simulink model "Copy_of_EIRSAT_ADCS"  (R2014a)
settings: Solver=ode45  SolverMode=SingleTasking  StartTime=0.0  StopTime=5900*5  FixedStep=1e-9  RelTol=1e-6
values from neighbouring files (symbols this model uses):
  adr = ADRblockGen(w,m,3)    [Control_mission_def.m]    (also in CubeSimSetUp.m; Example__simulaltion.m; Example_simulaltion.m; WBC_setup.m)
  adr2 = ADRblockGen(wo2,I(2,2),3)    [CubeQuat_setup.m]    (also in WBC_setup.m = ADRblockGen(w2,m,3))
  aerodrag_A_d = 0.2*0.1*sqrt(2)    [Satellite_Setup_Sun_Pointing.m]    (also in Satellite_setup_ZenithPointing.m; WS_20_09_2017.mat = 0.0282842712475; WS_25_09_2017.mat = 0.0282842712475; WS_29_09_2017.mat = 0.0282842712475)
  aerodrag_c_p = 0.02*[1;1;1]    [Satellite_Setup_Sun_Pointing.m]    (also in Satellite_setup_ZenithPointing.m; WS_20_09_2017.mat = [0.02 0.02 0.02]; WS_25_09_2017.mat = [0.02 0.02 0.02]; WS_29_09_2017.mat = [0.02 0.02 0.02])
  distrej = 0    [Control_mission_def.m]    (also in CubeSimSetUp.m; Example__simulaltion.m; Example_simulaltion.m; WBC_setup.m = 1)
  I = diag(I_mom) + [0 I_prd(1) I_prd(2); I_prd(1) 0 I_prd(3); I_prd(2) I_prd(3) 0]    [CubeQuat_setup.m]    (also in CubeSatModel.m = reshape(I,3,3); CubeSatSfun.m = block.DialogPrm(2).Data; CubeSimSetUp.m = diag([Ixx;Iyy;Izz]); Satellite_Setup.m = diag([Ixx;Iyy;Izz]))
  igrf_G = [-29619.4 -3401.55 3349 4078.8125 -1723.05 1043.83125 2118.1875 1226.671875 474.8046875 -469.10703125 930.012890625 -1452.42753906 ... (182 elements, 13x14)]    [WS_20_09_2017.mat]    (also in WS_25_09_2017.mat; WS_29_09_2017.mat)
  igrf_H = [0 0 0 0 0 0 0 0 0 0 0 0 ... (182 elements, 13x14)]    [WS_20_09_2017.mat]    (also in WS_25_09_2017.mat; WS_29_09_2017.mat)
  igrf_L = 10    [Satellite_Setup_Sun_Pointing.m]    (also in Satellite_setup_ZenithPointing.m; WS_20_09_2017.mat; WS_25_09_2017.mat; WS_29_09_2017.mat)
  igrf_tol = 1e-9    (= 1e-09)    [Satellite_Setup_Sun_Pointing.m]    (also in Satellite_setup_ZenithPointing.m; WS_20_09_2017.mat; WS_25_09_2017.mat; WS_29_09_2017.mat)
  k = 1e-9    (= 1e-09)    [Control_mission_def.m]    (also in CubeSimSetUp.m = 1e-06; Example__simulaltion.m; Example_simulaltion.m = 5e-08; WBC_setup.m = 5e-09)
  k2 = 10    [CubeQuat_setup.m]    (also in WBC_setup.m = 5e-09; WS_20_09_2017.mat = 5e-09; WS_25_09_2017.mat = 5e-09; WS_29_09_2017.mat = 1.56433333333e-08)
  k_bd = 1e-12    [WS_20_09_2017.mat]    (also in WS_25_09_2017.mat)
  kd = 6e-4    (= 0.0006)    [Control_mission_def.m]    (also in CubeQuat_setup.m = 2*sqrt(I(1,1))*sqrt(kp); CubeSimSetUp.m; Example__simulaltion.m; Example_simulaltion.m)
  kp = 5e-9    (= 5e-09)    [Control_mission_def.m]    (also in CubeQuat_setup.m = 40; CubeSimSetUp.m; Example__simulaltion.m; Example_simulaltion.m)
  mass = 15    [CubeQuat_setup.m]    (also in CubeSimSetUp.m = 2.6; Satellite_Setup.m = 2.6; Satellite_Setup_Sun_Pointing.m = 2.6; Satellite_setup_ZenithPointing.m = 2.6)
  nA = [nAx;nAy;nAz]    [Control_mission_def.m]    (also in WS_20_09_2017.mat = [0.48 0.48 0.48]; WS_25_09_2017.mat = [0.48 0.48 0.48]; WS_29_09_2017.mat = [0.48 0.48 0.48])
  omega_orbit = [0;-7.67/(401.1+6371);0]    [CubeQuat_setup.m]    (also in CubeSatModel.m = inputs(28:30); CubeSatSfun.m = block.DialogPrm(3).Data; CubeSimSetUp.m; Satellite_Setup.m)
  q_ref = q_3_ref    [Control_mission_def.m]    (also in CubeSimSetUp.m = angle2quat(0,0,0,'XYZ'); Example__simulaltion.m; Example_simulaltion.m; WS_20_09_2017.mat = [0.707106781187 0.707106781187 0 0])
  x_0 = [0,0,0,1,0,0,0]    [CubeQuat_setup.m]    (also in CubeSimSetUp.m = [wb_bi_init;qb_o_init;qb_i_init;qo_i_init;long_init;lat_init; Example__simulaltion.m = transpose([wb_bi_init,qb_i_init]); Example_simulaltion.m = transpose([wb_bi_init,qb_i_init]); Satellite_Setup.m = transpose([wb_bi_init,qb_i_init]))
  x_orbit_init = [long_init,lat_init,altitude,qb_o_init,qo_i_init]    [Example__simulaltion.m]    (also in Example_simulaltion.m; Satellite_Setup.m; Satellite_Setup_Sun_Pointing.m; Satellite_setup_ZenithPointing.m)
undefined symbols (not defined in the file or in its folder): i_coil, m_coil, sfunxyz, SkewSym, T_act
libraries: cstblocks x24, aerolibtransform2 x7, vrlib x6
(part 1 of 2)
settings Model: Creator=JoeT  LastModifiedBy=Daire
settings OptimizationCC: BlockReduction=off  BooleanDataType=off
settings DebuggingCC: SaveWithParameterizedLinksMsg=none  UnderspecifiedInitializationDetection=Classic  SignalResolutionControl=TryResolveAllWithWarning  SolverPrmCheckMsg=none
settings HardwareCC: TargetUnknown=on

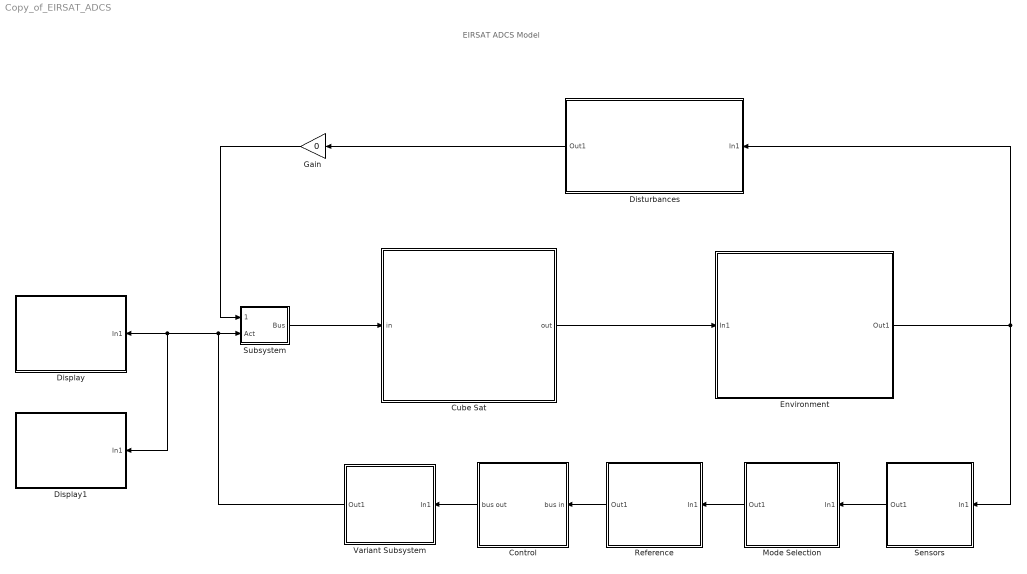
== system Copy_of_EIRSAT_ADCS ==
  note: EIRSAT ADCS Model
  Control : Subsystem  Variant=on
  Cube Sat : Subsystem
  Display : Subsystem
  Display1 : Subsystem
  Disturbances : Subsystem
  Environment : Subsystem
  Gain : Gain  Gain=0
  Mode Selection : Subsystem
  Reference : Subsystem
  Sensors : Subsystem
  Subsystem : Subsystem
  Variant Subsystem : Subsystem  Variant=on
  wires:
  Mode Selection/1(Out1) -> Reference/1(In1)
  Sensors/1(Out1) -> Mode Selection/1(In1)
  Reference/1(Out1) -> Control/1(bus in)
  Control/1(bus out) -> Variant Subsystem/1(In1)
  Disturbances/1(Out1) -> Gain/1
  Cube Sat/1(out) -> Environment/1(In1)
  Environment/1(Out1) -> Sensors/1(In1), Disturbances/1(In1)
  Variant Subsystem/1(Out1) -> Subsystem/2(Act), Display1/1(In1), Display/1(In1)
  Subsystem/1(Bus) -> Cube Sat/1(in)
  Gain/1 -> Subsystem/1(Disturb)

== system Copy_of_EIRSAT_ADCS/Control ==
  note: 1) Only subsystems can be added as variant choices at this level
      | 2) Blocks cannot be connected at this level as connectivity is
      | automatically determined at simulation, based on the active variant
  bus in : Inport
  B dot : Subsystem  VariantControl=CtrlType==4
  PD : Subsystem  VariantControl=CtrlType==2
  PD Zenith : Subsystem  VariantControl=CtrlType==3
  WBC : Subsystem  VariantControl=CtrlType==1
  WBC detumble : Subsystem  VariantControl=CtrlType==5
  no control : Subsystem  VariantControl=CtrlType==0
  bus out : Outport

== system Copy_of_EIRSAT_ADCS/Cube Sat ==
  in : Inport
  Bus Creator : BusCreator  Inputs=8
  Bus Selector1 : BusSelector  OutputSignals=T_total,T_act
  Constant : Constant  Value=omega_orbit
  Constant1 : Constant  Value=[0;0;0]
  Gain : Gain
  Gain1 : Gain
  Level-2 MATLAB S-Function : M-S-Function  FunctionName=OrbitSfun  Parameters=x_orbit_init,omega_orbit  mask{Parameter1=x_orbit_init, Parameter2=omega_orbit}
      mask prompts: Parameter1 "Initial orbit param"; Parameter2 "orbit angular velocity"
      mask DialogControl Control8 Prompt: Orbit properties
      mask Display:
      | disp('Orbital Parameters')
      | port_label('input',1,'ang vel')
      | port_label('output',1,'LLA')
      | port_label('output',2,'qb_o')
      | port_label('output',3,'qo_i')
  Satellite Dyn : M-S-Function  FunctionName=CubeSatSfun  Parameters=x_0,I  mask{Parameter2=x_0, Parameter3=I}
      mask prompts: Parameter2 "x_0"; Parameter3 "I"
      mask DialogControl DescTextVar Prompt: Model of a rigid CubeSat. Model takes Torque about each axis as an input. The first output is the angular velocity of the sat wrt an inertial frame. The second output is the quaternion which represents the rotation between inertial and body fixed frames
      mask Display:
      | disp('Cube Sat Model')
      | port_label('input',1,'Torq')
      | port_label('output',1,'Ang Vel')
      | port_label('output',2,'Quat')
  Scope : Scope
      settings: SaveName=ScopeData15
  out : Outport
  wires:
  Bus Selector1/1 -> Gain/1  "<T_total>"
  Satellite Dyn/1 -> Level-2 MATLAB S-Function/1, Bus Creator/1  "omega_b_inert"
  Gain/1 -> Satellite Dyn/1, Scope/1
  Satellite Dyn/2 -> Bus Creator/2  "qb_i"
  Level-2 MATLAB S-Function/1 -> Bus Creator/3  "LongLatAlt"
  Level-2 MATLAB S-Function/2 -> Bus Creator/4  "qb_o"
  Level-2 MATLAB S-Function/3 -> Bus Creator/5  "qo_i"
  Constant/1 -> Bus Creator/7  "omega_orbit"
  Bus Selector1/2 -> Gain1/1  "<T_act>"
  Gain1/1 -> Bus Creator/6  "T_ctrlr"
  Constant1/1 -> Bus Creator/8  "B_i"
  in/1 -> Bus Selector1/1
  Bus Creator/1 -> out/1

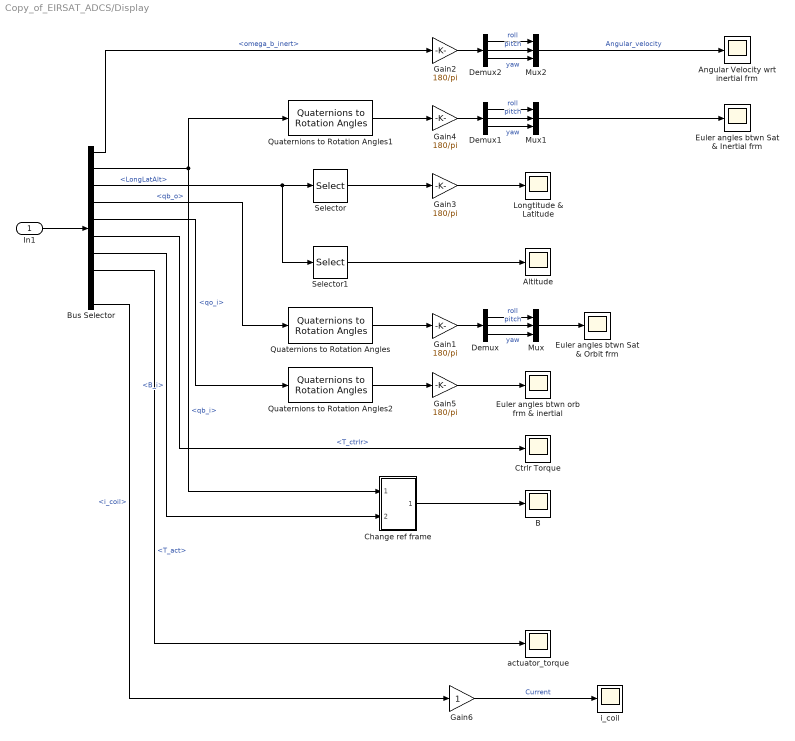
== system Copy_of_EIRSAT_ADCS/Display ==
  In1 : Inport
  Altitude : Scope
  Angular Velocity wrt inertial frm : Scope
      settings: ShowLegends=on  TimeRange=5445.680459835854  YMin=-0.3  YMax=1.1  SaveName=ScopeData5
  B : Scope
  Bus Selector : BusSelector  OutputSignals=Actual_Values.omega_b_inert,Actual_Values.qb_i,Actual_Values.LongLatAlt,Actual_Values.qb_o,Actual_Values.qo_i,Actual_Values.T_ctrlr,Actual_Values.B_i,T_act,q_ref,i_coil
  Change ref frame : Subsystem
  Ctrlr Torque : Scope
      settings: YMin=-5e-11  YMax=1.75e-10
  Demux : Demux  Outputs=3
  Demux1 : Demux  Outputs=3
  Demux2 : Demux  Outputs=3
  Euler angles btwn Sat & Inertial frm : Scope
      settings: ShowLegends=on  TimeRange=5655.978629419876  YMin=-3  YMax=4  SaveName=ScopeData8
  Euler angles btwn Sat & Orbit frm : Scope
      settings: ShowLegends=on  TimeRange=5445.680459835854  YMax=0.25
  Euler angles btwn orb frm & inertial : Scope
      settings: YMin=-200  YMax=100
  Gain{1..5} (5 alike) : Gain  Gain=180/pi
  Gain6 : Gain
  Longtitude & Latitude : Scope
  Mux : Mux  Inputs=3
  Mux1 : Mux  Inputs=3
  Mux2 : Mux  Inputs=3
  Quaternions to Rotation Angles : aerolibtransform2/Quaternions to Rotation Angles  rotationOrder=XYZ
  Quaternions to Rotation Angles1 : aerolibtransform2/Quaternions to Rotation Angles  rotationOrder=XYZ
  Quaternions to Rotation Angles2 : aerolibtransform2/Quaternions to Rotation Angles  rotationOrder=XYZ
  Selector : Selector  InputPortWidth=3  Indices=[1 2]
  Selector1 : Selector  InputPortWidth=3  Indices=[3]
  actuator_torque : Scope
      settings: YMin=-3.5e-09  YMax=2e-09
  i_coil : Scope
      settings: TimeRange=5445.680459835854  YMin=-0.001  YMax=0.0005  SaveName=ScopeData9
  wires:
  In1/1 -> Bus Selector/1
  Bus Selector/6 -> Ctrlr Torque/1  "<T_ctrlr>"
  Bus Selector/4 -> Quaternions to Rotation Angles/1  "<qb_o>"
  Bus Selector/1 -> Gain2/1  "<omega_b_inert>"
  Quaternions to Rotation Angles/1 -> Gain1/1
  Gain1/1 -> Demux/1
  Selector/1 -> Gain3/1
  Gain3/1 -> Longtitude & Latitude/1
  Bus Selector/2 -> Change ref frame/1(In1), Quaternions to Rotation Angles1/1  "<qb_i>"
  Quaternions to Rotation Angles1/1 -> Gain4/1
  Selector1/1 -> Altitude/1
  Bus Selector/5 -> Quaternions to Rotation Angles2/1  "<qo_i>"
  Quaternions to Rotation Angles2/1 -> Gain5/1
  Bus Selector/3 -> Selector1/1, Selector/1  "<LongLatAlt>"
  Bus Selector/8 -> actuator_torque/1  "<T_act>"
  Bus Selector/10 -> Gain6/1  "<i_coil>"
  Gain5/1 -> Euler angles btwn orb frm & inertial/1
  Demux/1 -> Mux/1  "roll"
  Demux/2 -> Mux/2  "pitch"
  Demux/3 -> Mux/3  "yaw"
  Mux/1 -> Euler angles btwn Sat & Orbit frm/1
  Demux1/1 -> Mux1/1  "roll"
  Demux1/2 -> Mux1/2  "pitch"
  Demux1/3 -> Mux1/3  "yaw"
  Gain4/1 -> Demux1/1
  Demux2/1 -> Mux2/1  "roll"
  Demux2/2 -> Mux2/2  "pitch"
  Demux2/3 -> Mux2/3  "yaw"
  Gain2/1 -> Demux2/1
  Mux2/1 -> Angular Velocity wrt inertial frm/1  "Angular_velocity"
  Gain6/1 -> i_coil/1  "Current"
  Mux1/1 -> Euler angles btwn Sat & Inertial frm/1
  Bus Selector/7 -> Change ref frame/2(In2)  "<B_i>"
  Change ref frame/1(Out1) -> B/1

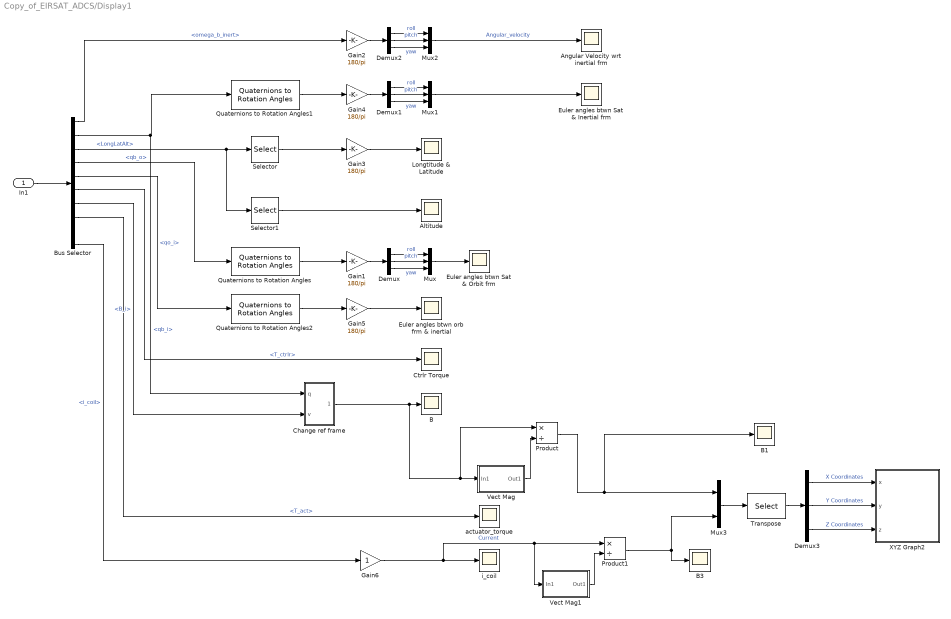
== system Copy_of_EIRSAT_ADCS/Display1 ==
  In1 : Inport
  Altitude : Scope
  Angular Velocity wrt inertial frm : Scope
      settings: ShowLegends=on  TimeRange=5445.680459835854  YMin=-0.3  YMax=1.1  SaveName=ScopeData5
  B : Scope
      settings: YMin=-2.25e-05  YMax=1.25e-05
  B1 : Scope
      settings: YMin=-0.9  YMax=0.5  SaveName=ScopeData3
  B3 : Scope
      settings: YMin=-1  YMax=0.2  SaveName=ScopeData6
  Bus Selector : BusSelector  OutputSignals=Actual_Values.omega_b_inert,Actual_Values.qb_i,Actual_Values.LongLatAlt,Actual_Values.qb_o,Actual_Values.qo_i,Actual_Values.T_ctrlr,Actual_Values.B_i,T_act,q_ref,i_coil
  Change ref frame : Subsystem
  Ctrlr Torque : Scope
      settings: YMin=-5e-11  YMax=1.75e-10
  Demux : Demux  Outputs=3
  Demux1 : Demux  Outputs=3
  Demux2 : Demux  Outputs=3
  Demux3 : Demux  Outputs=[2 2 2]
  Euler angles btwn Sat & Inertial frm : Scope
      settings: ShowLegends=on  TimeRange=5655.978629419876  YMin=-3  YMax=4  SaveName=ScopeData8
  Euler angles btwn Sat & Orbit frm : Scope
      settings: ShowLegends=on  TimeRange=5445.680459835854  YMax=0.25
  Euler angles btwn orb frm & inertial : Scope
      settings: YMin=-200  YMax=100
  Gain{1..5} (5 alike) : Gain  Gain=180/pi
  Gain6 : Gain
  Longtitude & Latitude : Scope
  Mux : Mux  Inputs=3
  Mux1 : Mux  Inputs=3
  Mux2 : Mux  Inputs=3
  Mux3 : Mux  Inputs=2
  Product : Product  Inputs=*/
  Product1 : Product  Inputs=*/
  Quaternions to Rotation Angles : aerolibtransform2/Quaternions to Rotation Angles  rotationOrder=XYZ
  Quaternions to Rotation Angles1 : aerolibtransform2/Quaternions to Rotation Angles  rotationOrder=XYZ
  Quaternions to Rotation Angles2 : aerolibtransform2/Quaternions to Rotation Angles  rotationOrder=XYZ
  Selector : Selector  InputPortWidth=3  Indices=[1 2]
  Selector1 : Selector  InputPortWidth=3  Indices=[3]
  Transpose : Selector  InputPortWidth=3*2  Indices=reshape(reshape(1:3*2,3,2)',3*2,1)
  Vect Mag : Subsystem
  Vect Mag1 : Subsystem
  XYZ Graph2 : Subsystem  LoadFcn=sfunxyz([],[],[],'LoadBlock')  StartFcn=sfunxyz([],[],[],'Start')  StopFcn=sfunxyz([],[],[],'Stop')  mask(XYZ multiscope){np=2, xlim=[-1 1], ylim=[-1 1], zlim=[-1 1], cp=[3 2 1], gd=on, st=0.1}
      mask prompts: np "Number of lines"; xlim "[xmin xmax]"; ylim "[ymin ymax]"; zlim "[zmin zmax]"; cp "Camera position (use [0 0 1] for 2D XY view)"; gd "Grid"; st "Sample time:"
      mask help:
      | Multidimensional XYZ scope using MATLAB graph window.
      |    X,Y,Z coordinates are respectively the first,second, and third input.
      |    Enter the number of lines, the XYZ ranges, the camera position,
      |    and the sampling time, as mask parameters.
      settings: CopyFcn=sfunxyz([],[],[],'CopyBlock')  DeleteFcn=sfunxyz([],[],[],'DeleteBlock')  NameChangeFcn=sfunxyz([],[],[],'NameChange')
      mask Help:
      | This block can be used to explore limit cycles.
      |    Look at the m-file sfunxyz.m to see how it works.
      mask Display: plot([.05 .95 .95 .05 .05],[.45 .45 .95 .95 .45], 0.5+cos(0:0.1:2*pi)*0.3,0.7+sin(0:0.1:2*pi)*0.2)
  actuator_torque : Scope
      settings: YMin=-3.5e-09  YMax=2e-09
  i_coil : Scope
      settings: TimeRange=5445.680459835854  YMin=-4.75e-06  YMax=7.5e-07  SaveName=ScopeData9
  wires:
  Change ref frame/1(Out1) -> Product/1, Vect Mag/1(In1), B/1
  Bus Selector/7 -> Change ref frame/2(v)  "<B_i>"
  Mux1/1 -> Euler angles btwn Sat & Inertial frm/1
  Gain6/1 -> Product1/1, Vect Mag1/1(In1), i_coil/1  "Current"
  Mux2/1 -> Angular Velocity wrt inertial frm/1  "Angular_velocity"
  Gain2/1 -> Demux2/1
  Demux2/3 -> Mux2/3  "yaw"
  Demux2/2 -> Mux2/2  "pitch"
  Demux2/1 -> Mux2/1  "roll"
  Gain4/1 -> Demux1/1
  Demux1/3 -> Mux1/3  "yaw"
  Demux1/2 -> Mux1/2  "pitch"
  Demux1/1 -> Mux1/1  "roll"
  Mux/1 -> Euler angles btwn Sat & Orbit frm/1
  Demux/3 -> Mux/3  "yaw"
  Demux/2 -> Mux/2  "pitch"
  Demux/1 -> Mux/1  "roll"
  Gain5/1 -> Euler angles btwn orb frm & inertial/1
  Bus Selector/10 -> Gain6/1  "<i_coil>"
  Bus Selector/8 -> actuator_torque/1  "<T_act>"
  Bus Selector/3 -> Selector/1, Selector1/1  "<LongLatAlt>"
  Quaternions to Rotation Angles2/1 -> Gain5/1
  Bus Selector/5 -> Quaternions to Rotation Angles2/1  "<qo_i>"
  Selector1/1 -> Altitude/1
  Quaternions to Rotation Angles1/1 -> Gain4/1
  Bus Selector/2 -> Quaternions to Rotation Angles1/1, Change ref frame/1(q)  "<qb_i>"
  Gain3/1 -> Longtitude & Latitude/1
  Selector/1 -> Gain3/1
  Gain1/1 -> Demux/1
  Quaternions to Rotation Angles/1 -> Gain1/1
  Bus Selector/1 -> Gain2/1  "<omega_b_inert>"
  Bus Selector/4 -> Quaternions to Rotation Angles/1  "<qb_o>"
  Bus Selector/6 -> Ctrlr Torque/1  "<T_ctrlr>"
  In1/1 -> Bus Selector/1
  Mux3/1 -> Transpose/1
  Transpose/1 -> Demux3/1
  Demux3/1 -> XYZ Graph2/1(x)  "X Coordinates"
  Demux3/2 -> XYZ Graph2/2(y)  "Y Coordinates"
  Demux3/3 -> XYZ Graph2/3(z)  "Z Coordinates"
  Vect Mag/1(Out1) -> Product/2
  Product/1 -> B1/1, Mux3/1
  Vect Mag1/1(Out1) -> Product1/2
  Product1/1 -> Mux3/2, B3/1

== system Copy_of_EIRSAT_ADCS/Disturbances ==
  In1 : Inport
  Bus Selector : BusSelector  OutputSignals=qb_o,omega_orbit,omega_b_inert
  Constant : Constant  Value=7.2157
  Level-2 MATLAB S-Function : M-S-Function  FunctionName=gravityGradientSfun
      mask Display:
      | disp('Gravity\n gradient')
      | port_label('input',1,'qb_o')
      | port_label('input',2,'omega orbit')
      | port_label('output',1,'T_b')
  Level-2 MATLAB S-Function1 : M-S-Function  FunctionName=aeroDragSfun  Parameters=I,mass,aerodrag_c_p,aerodrag_A_d  mask{Parameter1=I, Parameter2=mass, Parameter3=aerodrag_c_p, Parameter4=aerodrag_A_d}
      mask prompts: Parameter1 "Inertia"; Parameter2 "Mass"; Parameter3 "COP vector"; Parameter4 "Area"
      mask Display:
      | disp('Aerodynamic\n drag')
      | port_label('input',1,'qb_o')
      | port_label('input',2,'omega orbit')
      | port_label('input',3,'Local atmosph. vel')
      | port_label('output',1,'T_b')
  Sum : Sum  Inputs=|++
  Out1 : Outport
  wires:
  Level-2 MATLAB S-Function/1 -> Sum/1
  Level-2 MATLAB S-Function1/1 -> Sum/2
  In1/1 -> Bus Selector/1
  Bus Selector/1 -> Level-2 MATLAB S-Function1/1, Level-2 MATLAB S-Function/1  "<qb_o>"
  Bus Selector/2 -> Level-2 MATLAB S-Function/2, Level-2 MATLAB S-Function1/2  "<omega_orbit>"
  Constant/1 -> Level-2 MATLAB S-Function1/3
  Sum/1 -> Out1/1  "T_dst"
  Bus Selector/3 -> Level-2 MATLAB S-Function1/4  "<omega_b_inert>"

== system Copy_of_EIRSAT_ADCS/Environment ==
  In1 : Inport
  Bus Assignment : BusAssignment  AssignedSignals=B_i
  Bus Selector : BusSelector  OutputSignals=LongLatAlt
  Constant : Constant  Value=0
  Level-2 MATLAB S-Function : M-S-Function  FunctionName=IGRFSfun  Parameters=igrf_L,igrf_tol,igrf_G,igrf_H  mask{Parameter1=igrf_L, Parameter2=igrf_tol, Parameter3=igrf_G, Parameter4=igrf_H}
      mask prompts: Parameter1 "L"; Parameter2 "tolerance"; Parameter3 "G_coefs"; Parameter4 "H_coefs"
      mask Display:
      | disp('IGRF 11\n  Geomagnetic reference')
      | port_label('input',1,'LLA')
      | port_label('output',1,'real B')
  Out1 : Outport
  wires:
  In1/1 -> Bus Selector/1, Bus Assignment/1  "Dyn_out"
  Bus Selector/1 -> Level-2 MATLAB S-Function/1  "<LongLatAlt>"
  Bus Assignment/1 -> Out1/1
  Constant/1 -> Level-2 MATLAB S-Function/2  "B_real"
  Level-2 MATLAB S-Function/1 -> Bus Assignment/2  "B_real"

== system Copy_of_EIRSAT_ADCS/Mode Selection ==
  In1 : Inport
  Bus Assignment : BusAssignment  AssignedSignals=Mode
  Constant : Constant
  Out1 : Outport
  wires:
  In1/1 -> Bus Assignment/1  "Sensor_out"
  Bus Assignment/1 -> Out1/1
  Constant/1 -> Bus Assignment/2  "mode"

== system Copy_of_EIRSAT_ADCS/Reference ==
  In1 : Inport
  Bus Assignment : BusAssignment  AssignedSignals=q_ref
  Constant : Constant  Value=q_ref
  Out1 : Outport
  wires:
  In1/1 -> Bus Assignment/1
  Bus Assignment/1 -> Out1/1
  Constant/1 -> Bus Assignment/2  "q_ref"

== system Copy_of_EIRSAT_ADCS/Sensors ==
  In1 : Inport
  Bus Creator1 : BusCreator  Inputs=10
  Bus Selector : BusSelector  OutputSignals=B_i,LongLatAlt,qb_i,omega_b_inert  OutputAsBus=on
  Constant : Constant
  Constant1 : Constant  Value=[1,0,0,0]
  Constant{2..7} (6 alike) : Constant  Value=[0;0;0]
  Out1 : Outport
  wires:
  In1/1 -> Bus Creator1/1, Bus Selector/1  "Actual_Values"
  Bus Creator1/1 -> Out1/1
  Bus Selector/1 -> Bus Creator1/2  "Sensor_Values"
  Constant/1 -> Bus Creator1/3  "Mode"
  Constant1/1 -> Bus Creator1/4  "q_ref"
  Constant2/1 -> Bus Creator1/5  "m_b"
  Constant3/1 -> Bus Creator1/6  "m_coil"
  Constant4/1 -> Bus Creator1/7  "T_act"
  Constant5/1 -> Bus Creator1/8  "i_coil"
  Constant6/1 -> Bus Creator1/9  "T_total"
  Constant7/1 -> Bus Creator1/10  "T_ctrlr"

== system Copy_of_EIRSAT_ADCS/Subsystem ==
  Disturb : Inport
  Act : Inport  Port=2
  Bus Assignment : BusAssignment  AssignedSignals=T_total
  Bus Selector1 : BusSelector  OutputSignals=T_act
  Sum : Sum  Inputs=++|
  Bus : Outport
  wires:
  Disturb/1 -> Sum/2
  Act/1 -> Bus Assignment/1, Bus Selector1/1
  Sum/1 -> Bus Assignment/2  "T_total"
  Bus Selector1/1 -> Sum/1  "<T_act>"
  Bus Assignment/1 -> Bus/1

== system Copy_of_EIRSAT_ADCS/Variant Subsystem ==
  note: 1) Only subsystems can be added as variant choices at this level
      | 2) Blocks cannot be connected at this level as connectivity is
      | automatically determined at simulation, based on the active variant
  In1 : Inport
  2 coil dipole : Subsystem  VariantControl=ActType==5
  3 coil dipole : Subsystem  VariantControl=ActType==4
  Ideal Torque : Subsystem  VariantControl=ActType==1
  No Torque : Subsystem  VariantControl=ActType==0
  Three Axis MagTorq : Subsystem  VariantControl=ActType==2
  Two Axis MagTorq : Subsystem  VariantControl=ActType==3
  Out1 : Outport

== system Copy_of_EIRSAT_ADCS/Control/B dot ==
  bus in : Inport
  Bus Creator : BusCreator  Inputs=2
  Bus Selector : BusSelector  OutputSignals=signal1.Sensor_out.Sensor_Values.qb_i,q_ref,signal1.Sensor_out.Sensor_Values.omega_b_inert,signal1.Sensor_out.Sensor_Values.B_real,signal1.Sensor_out.Actual_Values.Dyn_out.qb_o
  Derivative : Derivative
  Gain : Gain  Gain=-k_bd
  bus out : Outport
  wires:
  Bus Creator/1 -> bus out/1
  bus in/1 -> Bus Creator/1, Bus Selector/1  "ref_out"
  Bus Selector/4 -> Derivative/1  "<B_real>"
  Derivative/1 -> Gain/1
  Gain/1 -> Bus Creator/2  "T_ctrlr"

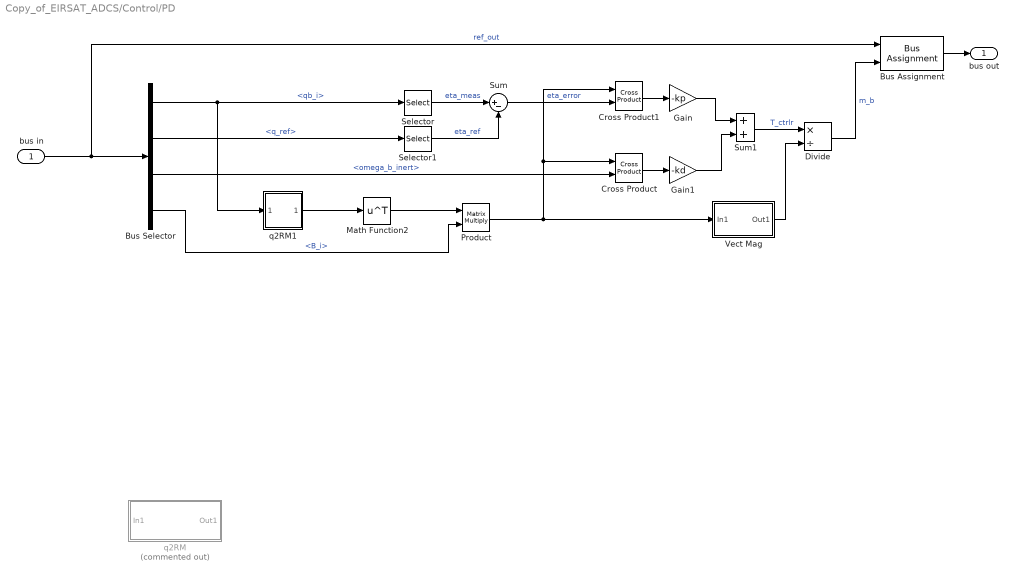
== system Copy_of_EIRSAT_ADCS/Control/PD ==
  bus in : Inport
  Bus Assignment : BusAssignment  AssignedSignals=m_b
  Bus Selector : BusSelector  OutputSignals=Sensor_Values.qb_i,q_ref,Sensor_Values.omega_b_inert,Sensor_Values.B_i
  Cross Product : vrlib/Utilities/Cross Product
  Cross Product1 : vrlib/Utilities/Cross Product
  Divide : Product  Inputs=*/
  Gain : Gain  Gain=-kp
  Gain1 : Gain  Gain=-kd
  Math Function2 : Math  Operator=transpose  SaturateOnIntegerOverflow=on
  Product : Product  Multiplication=Matrix(*)
  Selector : Selector  InputPortWidth=4  Indices=[2 3 4]
  Selector1 : Selector  InputPortWidth=4  Indices=[2 3 4]
  Sum : Sum  Inputs=|+-
  Sum1 : Sum
  Vect Mag : Subsystem
  q2RM : Subsystem  Commented=on
  q2RM1 : Subsystem
  bus out : Outport
  wires:
  bus in/1 -> Bus Assignment/1, Bus Selector/1  "ref_out"
  Bus Selector/2 -> Selector1/1  "<q_ref>"
  Selector/1 -> Sum/1  "eta_meas"
  Selector1/1 -> Sum/2  "eta_ref"
  Gain/1 -> Sum1/1
  Gain1/1 -> Sum1/2
  Bus Assignment/1 -> bus out/1
  Product/1 -> Cross Product1/1, Cross Product/1, Vect Mag/1(In1)
  Vect Mag/1(Out1) -> Divide/2
  Sum/1 -> Cross Product1/2  "eta_error"
  Bus Selector/1 -> q2RM1/1(In1), Selector/1  "<qb_i>"
  Cross Product1/1 -> Gain/1
  Cross Product/1 -> Gain1/1
  Divide/1 -> Bus Assignment/2  "m_b"
  Bus Selector/4 -> Product/2  "<B_i>"
  Math Function2/1 -> Product/1
  q2RM1/1(Out1) -> Math Function2/1
  Sum1/1 -> Divide/1  "T_ctrlr"
  Bus Selector/3 -> Cross Product/2  "<omega_b_inert>"

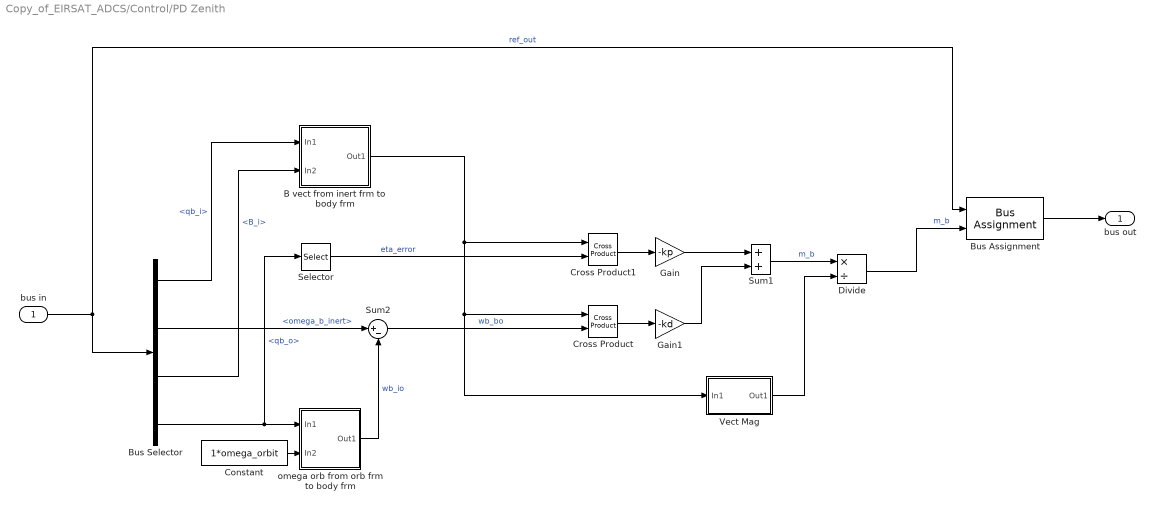
== system Copy_of_EIRSAT_ADCS/Control/PD Zenith ==
  bus in : Inport
  B vect from inert frm to body frm : Subsystem
  Bus Assignment : BusAssignment  AssignedSignals=m_b
  Bus Selector : BusSelector  OutputSignals=Sensor_Values.qb_i,Sensor_Values.omega_b_inert,Sensor_Values.B_i,Actual_Values.qb_o
  Constant : Constant  Value=1*omega_orbit
  Cross Product : vrlib/Utilities/Cross Product
  Cross Product1 : vrlib/Utilities/Cross Product
  Divide : Product  Inputs=*/
  Gain : Gain  Gain=-kp
  Gain1 : Gain  Gain=-kd
  Selector : Selector  InputPortWidth=4  Indices=[2 3 4]
  Sum1 : Sum
  Sum2 : Sum  Inputs=|+-
  Vect Mag : Subsystem
  omega orb from orb frm to body frm : Subsystem
  bus out : Outport
  wires:
  Divide/1 -> Bus Assignment/2  "m_b"
  Cross Product1/1 -> Gain/1
  Cross Product/1 -> Gain1/1
  Selector/1 -> Cross Product1/2  "eta_error"
  Sum1/1 -> Divide/1  "m_b"
  Sum2/1 -> Cross Product/2  "wb_bo"
  Vect Mag/1(Out1) -> Divide/2
  Bus Assignment/1 -> bus out/1
  Gain1/1 -> Sum1/2
  Gain/1 -> Sum1/1
  bus in/1 -> Bus Assignment/1, Bus Selector/1  "ref_out"
  Bus Selector/2 -> Sum2/1  "<omega_b_inert>"
  Bus Selector/4 -> Selector/1, omega orb from orb frm to body frm/1(In1)  "<qb_o>"
  Constant/1 -> omega orb from orb frm to body frm/2(In2)
  omega orb from orb frm to body frm/1(Out1) -> Sum2/2  "wb_io"
  B vect from inert frm to body frm/1(Out1) -> Vect Mag/1(In1), Cross Product/1, Cross Product1/1
  Bus Selector/1 -> B vect from inert frm to body frm/1(In1)  "<qb_i>"
  Bus Selector/3 -> B vect from inert frm to body frm/2(In2)  "<B_i>"

== system Copy_of_EIRSAT_ADCS/Control/WBC ==
  bus in : Inport
  Bus Assignment : BusAssignment  AssignedSignals=T_ctrlr
  Bus Selector : BusSelector  OutputSignals=q_ref,Sensor_Values.qb_i,Actual_Values.T_ctrlr,Sensor_Values.B_i
  Demux1 : Demux  Outputs=3
  Demux3 : Demux  Outputs=3
  Demux4 : Demux  Outputs=3
  Mux4 : Mux  Inputs=3
  Selector : Selector  InputPortWidth=4  Indices=[2 3 4]
  Selector1 : Selector  InputPortWidth=4  Indices=[2 3 4]
  WBC_x : Subsystem
  WBC_y : Subsystem
  WBC_z : Subsystem
  bus out : Outport
  wires:
  Demux3/3 -> WBC_z/2(x_1)
  WBC_y/1(T) -> Mux4/2
  Mux4/1 -> Bus Assignment/2  "T_ctrlr"
  WBC_z/1(T) -> Mux4/3
  WBC_x/1(T) -> Mux4/1
  Demux3/2 -> WBC_y/2(x_1)
  Demux3/1 -> WBC_x/2(x_1)
  Bus Selector/3 -> Demux1/1  "<T_ctrlr>"
  Demux1/1 -> WBC_x/3(T_meas)
  Demux1/2 -> WBC_y/3(T_meas)
  Demux1/3 -> WBC_z/3(T_meas)
  Demux4/1 -> WBC_x/1(x_0_ref)
  Demux4/3 -> WBC_z/1(x_0_ref)
  Demux4/2 -> WBC_y/1(x_0_ref)
  Selector1/1 -> Demux3/1
  bus in/1 -> Bus Assignment/1, Bus Selector/1  "ref_out"
  Bus Selector/1 -> Selector/1  "<q_ref>"
  Bus Selector/2 -> Selector1/1  "<qb_i>"
  Bus Assignment/1 -> bus out/1
  Selector/1 -> Demux4/1

== system Copy_of_EIRSAT_ADCS/Control/WBC detumble ==
  bus in : Inport
  Bus Creator : BusCreator  Inputs=2
  Bus Selector : BusSelector  OutputSignals=q_ref,signal1.Sensor_out.Sensor_values.omega_b_inert,signal1.Sensor_out.Enviro_out.Dyn_out.T_ctrlr
  Demux1 : Demux  Outputs=3
  Demux3 : Demux  Outputs=3
  Demux4 : Demux  Outputs=3
  Mux4 : Mux  Inputs=3
  Quaternions to Rotation Angles : aerolibtransform2/Quaternions to Rotation Angles  Commented=on  rotationOrder=ZYX
  Vector Mag1 : Subsystem  Commented=on
  WBC_x : Subsystem
  WBC_y : Subsystem
  WBC_z : Subsystem
  bus out : Outport
  wires:
  ? -> Demux4/1
  Bus Creator/1 -> bus out/1
  Bus Selector/2 -> Demux3/1  "<omega_b_inert>"
  Bus Selector/1 -> ?  "<q_ref>"
  bus in/1 -> Bus Selector/1, Bus Creator/1  "ref_out"
  Demux4/2 -> WBC_y/1(x_0_ref)
  Demux4/3 -> WBC_z/1(x_0_ref)
  Demux4/1 -> WBC_x/1(x_0_ref)
  Demux1/3 -> WBC_z/3(T_meas)
  Demux1/2 -> WBC_y/3(T_meas)
  Demux1/1 -> WBC_x/3(T_meas)
  Bus Selector/3 -> Demux1/1  "<T_ctrlr>"
  Demux3/1 -> WBC_x/2(x_1)
  Demux3/2 -> WBC_y/2(x_1)
  WBC_x/1(T) -> Mux4/1
  WBC_z/1(T) -> Mux4/3
  Mux4/1 -> Bus Creator/2  "T_ctrlr"
  WBC_y/1(T) -> Mux4/2
  Demux3/3 -> WBC_z/2(x_1)

== system Copy_of_EIRSAT_ADCS/Control/no control ==
  bus in : Inport
  Bus : Subsystem  Commented=on
  Bus Creator : BusCreator  Inputs=2
  Constant : Constant  Value=[0;0;0]
  bus out : Outport
  wires:
  bus in/1 -> Bus Creator/1  "ref_out"
  Constant/1 -> Bus Creator/2  "T_ctrlr"
  Bus Creator/1 -> bus out/1

== system Copy_of_EIRSAT_ADCS/Display/Change ref frame ==
  In1 : Inport
  In2 : Inport  Port=2
  Math Function2 : Math  Operator=transpose  SaturateOnIntegerOverflow=on
  Product : Product  Multiplication=Matrix(*)
  q2RM1 : Subsystem
  Out1 : Outport
  wires:
  Product/1 -> Out1/1
  Math Function2/1 -> Product/1
  In2/1 -> Product/2
  q2RM1/1(Out1) -> Math Function2/1
  In1/1 -> q2RM1/1(In1)

== system Copy_of_EIRSAT_ADCS/Display1/Change ref frame ==
  q : Inport
  v : Inport  Port=2
  Math Function2 : Math  Operator=transpose  SaturateOnIntegerOverflow=on
  Product : Product  Multiplication=Matrix(*)
  q2RM1 : Subsystem
  Out1 : Outport
  wires:
  q/1 -> q2RM1/1(In1)
  q2RM1/1(Out1) -> Math Function2/1
  v/1 -> Product/2
  Math Function2/1 -> Product/1
  Product/1 -> Out1/1

== system Copy_of_EIRSAT_ADCS/Display1/Vect Mag ==
  In1 : Inport
  Math Function : Math  Operator=square  SaturateOnIntegerOverflow=on
  Sqrt : Sqrt  SaturateOnIntegerOverflow=on
  Sum2 : Sum  Inputs=+
  Out1 : Outport
  wires:
  Sqrt/1 -> Out1/1
  In1/1 -> Math Function/1
  Math Function/1 -> Sum2/1
  Sum2/1 -> Sqrt/1

== system Copy_of_EIRSAT_ADCS/Display1/Vect Mag1 ==
  In1 : Inport
  Math Function : Math  Operator=square  SaturateOnIntegerOverflow=on
  Sqrt : Sqrt  SaturateOnIntegerOverflow=on
  Sum2 : Sum  Inputs=+
  Out1 : Outport
  wires:
  Sum2/1 -> Sqrt/1
  Math Function/1 -> Sum2/1
  In1/1 -> Math Function/1
  Sqrt/1 -> Out1/1

== system Copy_of_EIRSAT_ADCS/Display1/XYZ Graph2 ==
  x : Inport
  y : Inport  Port=2
  z : Inport  Port=3
  Mux : Mux  Inputs=[np np np]
  sfunxy : S-Function  FunctionName=sfunxyz  Parameters=[xlim ylim zlim],st,np,cp,gd  EnableBusSupport=off
  wires:
  z/1 -> Mux/3
  y/1 -> Mux/2
  x/1 -> Mux/1
  Mux/1 -> sfunxy/1

== system Copy_of_EIRSAT_ADCS/Variant Subsystem/2 coil dipole ==
  In1 : Inport
  B vect from inert frm to body frm : Subsystem
  Bus Assignment : BusAssignment  AssignedSignals=m_coil,T_act,i_coil
  Bus Selector : BusSelector  OutputSignals=m_b,Sensor_Values.B_i,Sensor_Values.qb_i
  Constant : Constant  Value=nA
  Constant3 : Constant  Value=0
  Cross Product : vrlib/Utilities/Cross Product
  Divide : Product  Inputs=*/
  Mux1 : Mux  Inputs=2
  Saturation : Saturate  UpperLimit=0.24  LowerLimit=-0.24
  Selector : Selector  InputPortWidth=3  Indices=[1 2]
  Out1 : Outport
  wires:
  Saturation/1 -> Bus Assignment/2, Divide/1, Cross Product/1
  Constant/1 -> Divide/2
  Divide/1 -> Bus Assignment/4  "i_coil"
  Bus Selector/1 -> Selector/1  "<m_b>"
  Cross Product/1 -> Bus Assignment/3  "T_act"
  Bus Assignment/1 -> Out1/1
  In1/1 -> Bus Selector/1, Bus Assignment/1  "Ctrlr_out"
  Mux1/1 -> Saturation/1
  Selector/1 -> Mux1/1
  Constant3/1 -> Mux1/2
  Bus Selector/2 -> B vect from inert frm to body frm/1(B_i)  "<B_i>"
  Bus Selector/3 -> B vect from inert frm to body frm/2(q)  "<qb_i>"
  B vect from inert frm to body frm/1(B_b) -> Cross Product/2

== system Copy_of_EIRSAT_ADCS/Variant Subsystem/3 coil dipole ==
  In1 : Inport
  B vect from inert frm to body frm : Subsystem
  Bus Assignment : BusAssignment  AssignedSignals=m_coil,T_act,i_coil
  Bus Selector : BusSelector  OutputSignals=m_b,Sensor_Values.B_i,Sensor_Values.qb_i
  Constant : Constant  Value=nA
  Cross Product : vrlib/Utilities/Cross Product
  Divide : Product  Inputs=*/
  Saturation : Saturate  UpperLimit=0.24  LowerLimit=-0.24
  Out1 : Outport
  wires:
  Saturation/1 -> Bus Assignment/2, Divide/1, Cross Product/1
  Constant/1 -> Divide/2
  Divide/1 -> Bus Assignment/4  "i_coil"
  Bus Selector/1 -> Saturation/1  "<m_b>"
  Cross Product/1 -> Bus Assignment/3  "T_act"
  In1/1 -> Bus Selector/1, Bus Assignment/1  "Ctrlr_out"
  Bus Selector/2 -> B vect from inert frm to body frm/1(B_i)  "<B_i>"
  Bus Selector/3 -> B vect from inert frm to body frm/2(q)  "<qb_i>"
  B vect from inert frm to body frm/1(B_b) -> Cross Product/2
  Bus Assignment/1 -> Out1/1

== system Copy_of_EIRSAT_ADCS/Variant Subsystem/Ideal Torque ==
  In1 : Inport
  Bus Creator : BusCreator  Inputs=3
  Bus Selector : BusSelector  OutputSignals=Actual_Values.T_ctrlr
  Constant : Constant  Value=[0,0,0]
  Gain : Gain
  Out1 : Outport
  wires:
  In1/1 -> Bus Selector/1, Bus Creator/1  "Ctrlr_out"
  Bus Creator/1 -> Out1/1
  Bus Selector/1 -> Gain/1  "<T_ctrlr>"
  Gain/1 -> Bus Creator/2  "T_act"
  Constant/1 -> Bus Creator/3  "i_coil"

== system Copy_of_EIRSAT_ADCS/Variant Subsystem/No Torque ==
  In1 : Inport
  Bus Assignment : BusAssignment  AssignedSignals=T_act,m_coil,i_coil
  Constant : Constant  Value=[0;0;0]
  Out1 : Outport
  wires:
  In1/1 -> Bus Assignment/1
  Bus Assignment/1 -> Out1/1
  Constant/1 -> Bus Assignment/4, Bus Assignment/3, Bus Assignment/2

== system Copy_of_EIRSAT_ADCS/Variant Subsystem/Three Axis MagTorq ==
  In1 : Inport
  B vect from inert frm to body frm : Subsystem
  B vect from inert frm to body frm1 : Subsystem
  Bus Assignment : BusAssignment  AssignedSignals=T_act,m_coil,i_coil
  Bus Selector : BusSelector  OutputSignals=T_ctrlr,Actual_Values.B_i,Sensor_Values.B_i,Sensor_Values.qb_i
  Level-2 MATLAB S-Function : M-S-Function  FunctionName=Magtorq2Sfun  Parameters=nAx, nAy, nAz
  Out1 : Outport
  wires:
  In1/1 -> Bus Assignment/1, Bus Selector/1
  Bus Assignment/1 -> Out1/1
  Bus Selector/3 -> Level-2 MATLAB S-Function/3, B vect from inert frm to body frm1/2(B_i)  "<B_i>"
  Level-2 MATLAB S-Function/1 -> Bus Assignment/2  "T_act"
  Bus Selector/1 -> Level-2 MATLAB S-Function/1  "<T_ctrlr>"
  Bus Selector/2 -> Level-2 MATLAB S-Function/2, B vect from inert frm to body frm/2(B_i)  "<B_i>"
  Level-2 MATLAB S-Function/2 -> Bus Assignment/3  "m_coil"
  Level-2 MATLAB S-Function/3 -> Bus Assignment/4  "i_coil"
  Bus Selector/4 -> B vect from inert frm to body frm1/1(q), B vect from inert frm to body frm/1(q)  "<qb_i>"
  B vect from inert frm to body frm/1(B_b) -> ?
  B vect from inert frm to body frm1/1(B_b) -> ?

== system Copy_of_EIRSAT_ADCS/Variant Subsystem/Two Axis MagTorq ==
  In1 : Inport
  Bus Creator : BusCreator
  Bus Selector : BusSelector  OutputSignals=T_ctrlr,ref_out.Mode_select_out.Sensor_out.Enviro_out.B_real,ref_out.Mode_select_out.Sensor_out.Sensor_values.B_real
  Level-2 MATLAB S-Function : M-S-Function  FunctionName=MagtorqSfun
  Selector : Selector  InputPortWidth=3  Indices=[1 2]
  Out1 : Outport
  wires:
  In1/1 -> Bus Selector/1, Bus Creator/1
  Bus Creator/1 -> Out1/1
  Bus Selector/3 -> Level-2 MATLAB S-Function/3  "<B_real>"
  Bus Selector/1 -> Level-2 MATLAB S-Function/1  "<T_ctrlr>"
  Bus Selector/2 -> Level-2 MATLAB S-Function/2  "<B_real>"
  Level-2 MATLAB S-Function/1 -> Selector/1
  Selector/1 -> Bus Creator/2  "m_coils"
  Level-2 MATLAB S-Function/2 -> Bus Creator/3
  ? -> Bus Creator/4  "i_coil"

== system Copy_of_EIRSAT_ADCS/Control/PD/Vect Mag ==
  In1 : Inport
  Math Function : Math  Operator=square  SaturateOnIntegerOverflow=on
  Sqrt : Sqrt  SaturateOnIntegerOverflow=on
  Sum2 : Sum  Inputs=+
  Out1 : Outport
  wires:
  Sqrt/1 -> Out1/1
  In1/1 -> Math Function/1
  Math Function/1 -> Sum2/1
  Sum2/1 -> Sqrt/1

== system Copy_of_EIRSAT_ADCS/Control/PD/q2RM ==
  In1 : Inport
  Add : Sum
  Constant : Constant  Value=eye(3)
  Fcn1 : Fcn  Expr=SkewSym([u(1),u(2),u(3)])
  Gain : Gain
  Math Function : Math  Operator=square  SaturateOnIntegerOverflow=on
  Product : Product
  Selector : Selector  InputPortWidth=4  Indices=[1]
  Selector1 : Selector  InputPortWidth=4  Indices=[2 3 4]
  Sum : Sum
  Out1 : Outport
  wires:
  In1/1 -> Selector/1, Selector1/1
  Fcn1/1 -> Math Function/1, Product/2
  Selector/1 -> Product/1
  Selector1/1 -> Fcn1/1
  Product/1 -> Sum/1
  Math Function/1 -> Sum/2
  Sum/1 -> Gain/1
  Gain/1 -> Add/2
  Constant/1 -> Add/1
  Add/1 -> Out1/1

== system Copy_of_EIRSAT_ADCS/Control/PD/q2RM1 ==
  In1 : Inport
  Add : Sum
  Constant : Constant  Value=eye(3)
  Fcn : Fcn  Commented=on  Expr=SkewSym([u(1),u(2),u(3)])
  Gain : Gain  Gain=2
  Interpreted MATLAB Function : MATLABFcn  MATLABFcn=SkewSym([u(1),u(2),u(3)],1)  OutputDimensions=9
  Math Function : Math  Operator=square  SaturateOnIntegerOverflow=on
  Product : Product
  Reshape : Reshape  OutputDimensionality=Customize  OutputDimensions=[3,3]
  Selector : Selector  InputPortWidth=4  Indices=[1]
  Selector1 : Selector  InputPortWidth=4  Indices=[2 3 4]
  Sum : Sum
  Out1 : Outport
  wires:
  In1/1 -> Selector/1, Selector1/1
  Reshape/1 -> Math Function/1, Product/2
  Selector/1 -> Product/1
  Selector1/1 -> Interpreted MATLAB Function/1
  Product/1 -> Sum/1
  Math Function/1 -> Sum/2
  Sum/1 -> Gain/1
  Gain/1 -> Add/2
  Constant/1 -> Add/1
  Add/1 -> Out1/1
  Interpreted MATLAB Function/1 -> Reshape/1

== system Copy_of_EIRSAT_ADCS/Control/PD Zenith/B vect from inert frm to body frm ==
  In1 : Inport
  In2 : Inport  Port=2
  Math Function1 : Math  Operator=transpose  SaturateOnIntegerOverflow=on
  Product1 : Product  Multiplication=Matrix(*)
  q2RM2 : Subsystem
  Out1 : Outport
  wires:
  Product1/1 -> Out1/1
  q2RM2/1(Out1) -> Math Function1/1
  In1/1 -> q2RM2/1(In1)
  Math Function1/1 -> Product1/1
  In2/1 -> Product1/2

== system Copy_of_EIRSAT_ADCS/Control/PD Zenith/Vect Mag ==
  In1 : Inport
  Math Function : Math  Operator=square  SaturateOnIntegerOverflow=on
  Sqrt : Sqrt  SaturateOnIntegerOverflow=on
  Sum2 : Sum  Inputs=+
  Out1 : Outport
  wires:
  Sum2/1 -> Sqrt/1
  Math Function/1 -> Sum2/1
  In1/1 -> Math Function/1
  Sqrt/1 -> Out1/1

== system Copy_of_EIRSAT_ADCS/Control/PD Zenith/omega orb from orb frm to body frm ==
  In1 : Inport
  In2 : Inport  Port=2
  Math Function2 : Math  Operator=transpose  SaturateOnIntegerOverflow=on
  Product : Product  Multiplication=Matrix(*)
  q2RM1 : Subsystem
  Out1 : Outport
  wires:
  Product/1 -> Out1/1
  In2/1 -> Product/2
  q2RM1/1(Out1) -> Math Function2/1
  Math Function2/1 -> Product/1
  In1/1 -> q2RM1/1(In1)

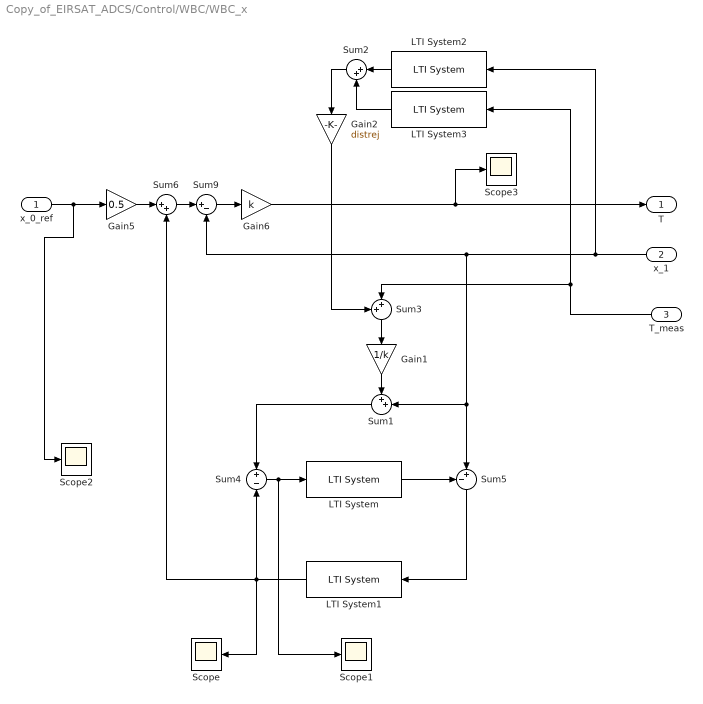
== system Copy_of_EIRSAT_ADCS/Control/WBC/WBC_x ==
  x_0_ref : Inport
  x_1 : Inport  Port=2
  T_meas : Inport  Port=3
  Gain1 : Gain  Gain=1/k
  Gain2 : Gain  Gain=distrej
  Gain5 : Gain  Gain=0.5
  Gain6 : Gain  Gain=k
  LTI System : cstblocks/LTI System  sys=G  IC=[]
  LTI System1 : cstblocks/LTI System  sys=G  IC=[]
  LTI System2 : cstblocks/LTI System  sys=adr(1)  IC=[]
  LTI System3 : cstblocks/LTI System  sys=adr(2)  IC=[]
  Scope{,1..3} (4 alike) : Scope
  Sum1 : Sum  Inputs=++|
  Sum2 : Sum  Inputs=|++
  Sum3 : Sum  Inputs=++|
  Sum4 : Sum  Inputs=+|-
  Sum5 : Sum  Inputs=-+|
  Sum6 : Sum  Inputs=|++
  Sum9 : Sum  Inputs=|+-
  T : Outport
  wires:
  Sum1/1 -> Sum4/1
  Gain1/1 -> Sum1/1
  x_1/1 -> Sum1/2, Sum5/2, Sum9/2, LTI System2/1
  Sum5/1 -> LTI System1/1
  LTI System/1 -> Sum5/1
  Sum4/1 -> Scope1/1, LTI System/1
  LTI System1/1 -> Sum4/2, Scope/1, Sum6/2
  Gain5/1 -> Sum6/1
  Gain6/1 -> Scope3/1, T/1
  Sum9/1 -> Gain6/1
  Sum6/1 -> Sum9/1
  LTI System2/1 -> Sum2/1
  LTI System3/1 -> Sum2/2
  Sum2/1 -> Gain2/1
  Sum3/1 -> Gain1/1
  Gain2/1 -> Sum3/1
  T_meas/1 -> Sum3/2, LTI System3/1
  x_0_ref/1 -> Scope2/1, Gain5/1

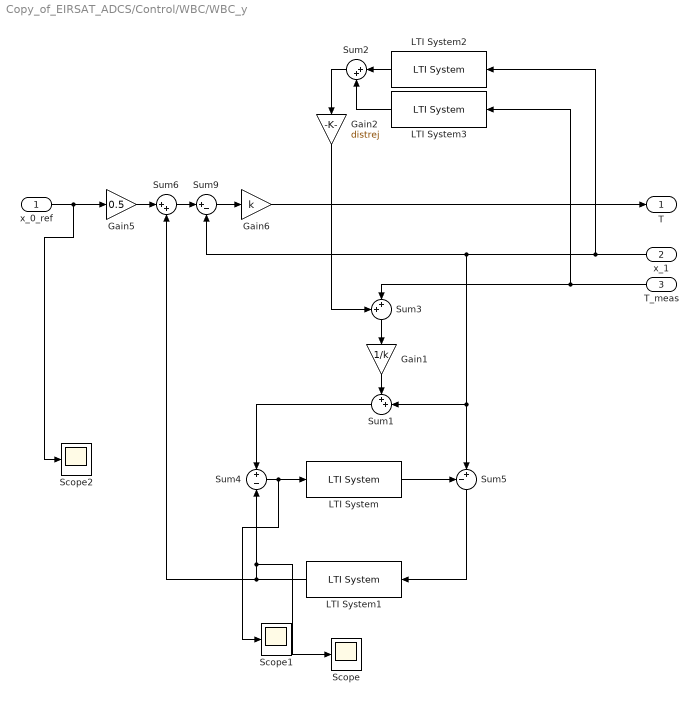
== system Copy_of_EIRSAT_ADCS/Control/WBC/WBC_y ==
  x_0_ref : Inport
  x_1 : Inport  Port=2
  T_meas : Inport  Port=3
  Gain1 : Gain  Gain=1/k
  Gain2 : Gain  Gain=distrej
  Gain5 : Gain  Gain=0.5
  Gain6 : Gain  Gain=k
  LTI System : cstblocks/LTI System  sys=G  IC=[]
  LTI System1 : cstblocks/LTI System  sys=G  IC=[]
  LTI System2 : cstblocks/LTI System  sys=adr(1)  IC=[]
  LTI System3 : cstblocks/LTI System  sys=adr(2)  IC=[]
  Scope : Scope
  Scope1 : Scope
  Scope2 : Scope
  Sum1 : Sum  Inputs=++|
  Sum2 : Sum  Inputs=|++
  Sum3 : Sum  Inputs=++|
  Sum4 : Sum  Inputs=+|-
  Sum5 : Sum  Inputs=-+|
  Sum6 : Sum  Inputs=|++
  Sum9 : Sum  Inputs=|+-
  T : Outport
  wires:
  x_0_ref/1 -> Gain5/1, Scope2/1
  T_meas/1 -> LTI System3/1, Sum3/2
  Gain2/1 -> Sum3/1
  Sum3/1 -> Gain1/1
  Sum2/1 -> Gain2/1
  LTI System3/1 -> Sum2/2
  LTI System2/1 -> Sum2/1
  Sum6/1 -> Sum9/1
  Sum9/1 -> Gain6/1
  Gain6/1 -> T/1
  Gain5/1 -> Sum6/1
  LTI System1/1 -> Sum6/2, Sum4/2, Scope/1
  Sum4/1 -> LTI System/1, Scope1/1
  LTI System/1 -> Sum5/1
  Sum5/1 -> LTI System1/1
  x_1/1 -> LTI System2/1, Sum9/2, Sum5/2, Sum1/2
  Gain1/1 -> Sum1/1
  Sum1/1 -> Sum4/1

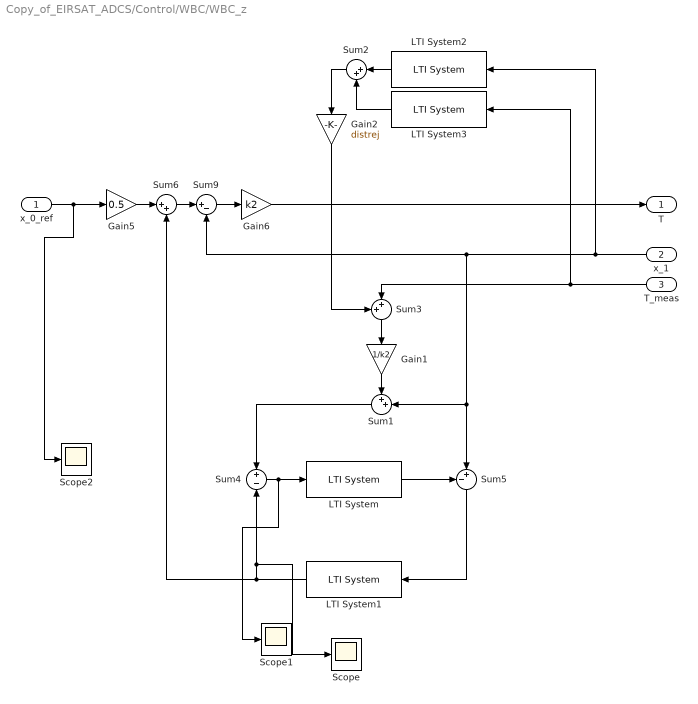
== system Copy_of_EIRSAT_ADCS/Control/WBC/WBC_z ==
  x_0_ref : Inport
  x_1 : Inport  Port=2
  T_meas : Inport  Port=3
  Gain1 : Gain  Gain=1/k2
  Gain2 : Gain  Gain=distrej
  Gain5 : Gain  Gain=0.5
  Gain6 : Gain  Gain=k2
  LTI System : cstblocks/LTI System  sys=G2  IC=[]
  LTI System1 : cstblocks/LTI System  sys=G2  IC=[]
  LTI System2 : cstblocks/LTI System  sys=adr2(1)  IC=[]
  LTI System3 : cstblocks/LTI System  sys=adr2(2)  IC=[]
  Scope : Scope
  Scope1 : Scope
  Scope2 : Scope
  Sum1 : Sum  Inputs=++|
  Sum2 : Sum  Inputs=|++
  Sum3 : Sum  Inputs=++|
  Sum4 : Sum  Inputs=+|-
  Sum5 : Sum  Inputs=-+|
  Sum6 : Sum  Inputs=|++
  Sum9 : Sum  Inputs=|+-
  T : Outport
  wires:
  Sum1/1 -> Sum4/1
  Gain1/1 -> Sum1/1
  x_1/1 -> Sum1/2, Sum5/2, Sum9/2, LTI System2/1
  Sum5/1 -> LTI System1/1
  LTI System/1 -> Sum5/1
  Sum4/1 -> Scope1/1, LTI System/1
  LTI System1/1 -> Scope/1, Sum4/2, Sum6/2
  Gain5/1 -> Sum6/1
  Gain6/1 -> T/1
  Sum9/1 -> Gain6/1
  Sum6/1 -> Sum9/1
  LTI System2/1 -> Sum2/1
  LTI System3/1 -> Sum2/2
  Sum2/1 -> Gain2/1
  Sum3/1 -> Gain1/1
  Gain2/1 -> Sum3/1
  T_meas/1 -> Sum3/2, LTI System3/1
  x_0_ref/1 -> Scope2/1, Gain5/1

== system Copy_of_EIRSAT_ADCS/Control/WBC detumble/Vector Mag1 ==
  v : Inport
  Math Function2 : Math  Operator=square  SaturateOnIntegerOverflow=on
  Sqrt2 : Sqrt  SaturateOnIntegerOverflow=on
  Sum2 : Sum  Inputs=+
  m : Outport
  wires:
  Sum2/1 -> Sqrt2/1
  Math Function2/1 -> Sum2/1
  v/1 -> Math Function2/1
  Sqrt2/1 -> m/1

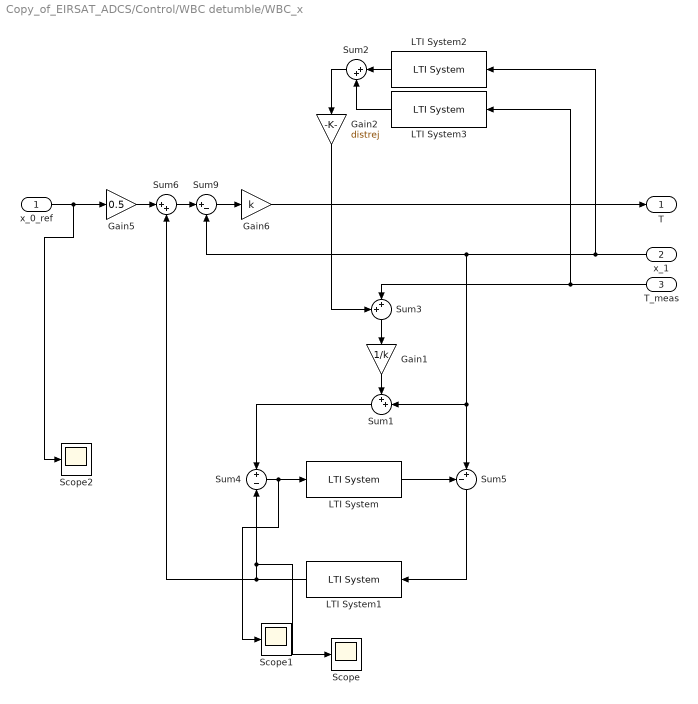
== system Copy_of_EIRSAT_ADCS/Control/WBC detumble/WBC_x ==
  x_0_ref : Inport
  x_1 : Inport  Port=2
  T_meas : Inport  Port=3
  Gain1 : Gain  Gain=1/k
  Gain2 : Gain  Gain=distrej
  Gain5 : Gain  Gain=0.5
  Gain6 : Gain  Gain=k
  LTI System : cstblocks/LTI System  sys=G  IC=[]
  LTI System1 : cstblocks/LTI System  sys=G  IC=[]
  LTI System2 : cstblocks/LTI System  sys=adr(1)  IC=[]
  LTI System3 : cstblocks/LTI System  sys=adr(2)  IC=[]
  Scope : Scope
  Scope1 : Scope
  Scope2 : Scope
  Sum1 : Sum  Inputs=++|
  Sum2 : Sum  Inputs=|++
  Sum3 : Sum  Inputs=++|
  Sum4 : Sum  Inputs=+|-
  Sum5 : Sum  Inputs=-+|
  Sum6 : Sum  Inputs=|++
  Sum9 : Sum  Inputs=|+-
  T : Outport
  wires:
  x_0_ref/1 -> Gain5/1, Scope2/1
  T_meas/1 -> LTI System3/1, Sum3/2
  Gain2/1 -> Sum3/1
  Sum3/1 -> Gain1/1
  Sum2/1 -> Gain2/1
  LTI System3/1 -> Sum2/2
  LTI System2/1 -> Sum2/1
  Sum6/1 -> Sum9/1
  Sum9/1 -> Gain6/1
  Gain6/1 -> T/1
  Gain5/1 -> Sum6/1
  LTI System1/1 -> Sum6/2, Sum4/2, Scope/1
  Sum4/1 -> LTI System/1, Scope1/1
  LTI System/1 -> Sum5/1
  Sum5/1 -> LTI System1/1
  x_1/1 -> LTI System2/1, Sum9/2, Sum5/2, Sum1/2
  Gain1/1 -> Sum1/1
  Sum1/1 -> Sum4/1

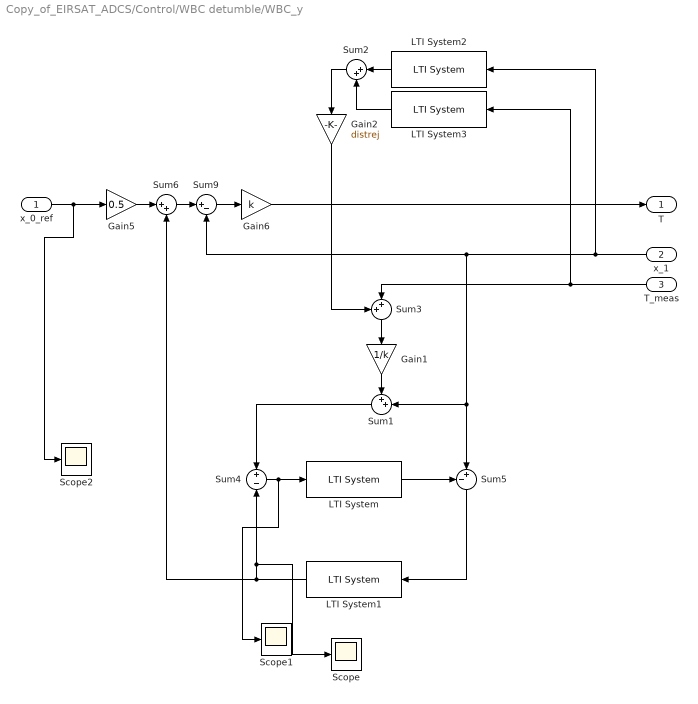
== system Copy_of_EIRSAT_ADCS/Control/WBC detumble/WBC_y ==
  x_0_ref : Inport
  x_1 : Inport  Port=2
  T_meas : Inport  Port=3
  Gain1 : Gain  Gain=1/k
  Gain2 : Gain  Gain=distrej
  Gain5 : Gain  Gain=0.5
  Gain6 : Gain  Gain=k
  LTI System : cstblocks/LTI System  sys=G  IC=[]
  LTI System1 : cstblocks/LTI System  sys=G  IC=[]
  LTI System2 : cstblocks/LTI System  sys=adr(1)  IC=[]
  LTI System3 : cstblocks/LTI System  sys=adr(2)  IC=[]
  Scope : Scope
  Scope1 : Scope
  Scope2 : Scope
  Sum1 : Sum  Inputs=++|
  Sum2 : Sum  Inputs=|++
  Sum3 : Sum  Inputs=++|
  Sum4 : Sum  Inputs=+|-
  Sum5 : Sum  Inputs=-+|
  Sum6 : Sum  Inputs=|++
  Sum9 : Sum  Inputs=|+-
  T : Outport
  wires:
  Sum1/1 -> Sum4/1
  Gain1/1 -> Sum1/1
  x_1/1 -> Sum1/2, Sum5/2, Sum9/2, LTI System2/1
  Sum5/1 -> LTI System1/1
  LTI System/1 -> Sum5/1
  Sum4/1 -> Scope1/1, LTI System/1
  LTI System1/1 -> Scope/1, Sum4/2, Sum6/2
  Gain5/1 -> Sum6/1
  Gain6/1 -> T/1
  Sum9/1 -> Gain6/1
  Sum6/1 -> Sum9/1
  LTI System2/1 -> Sum2/1
  LTI System3/1 -> Sum2/2
  Sum2/1 -> Gain2/1
  Sum3/1 -> Gain1/1
  Gain2/1 -> Sum3/1
  T_meas/1 -> Sum3/2, LTI System3/1
  x_0_ref/1 -> Scope2/1, Gain5/1

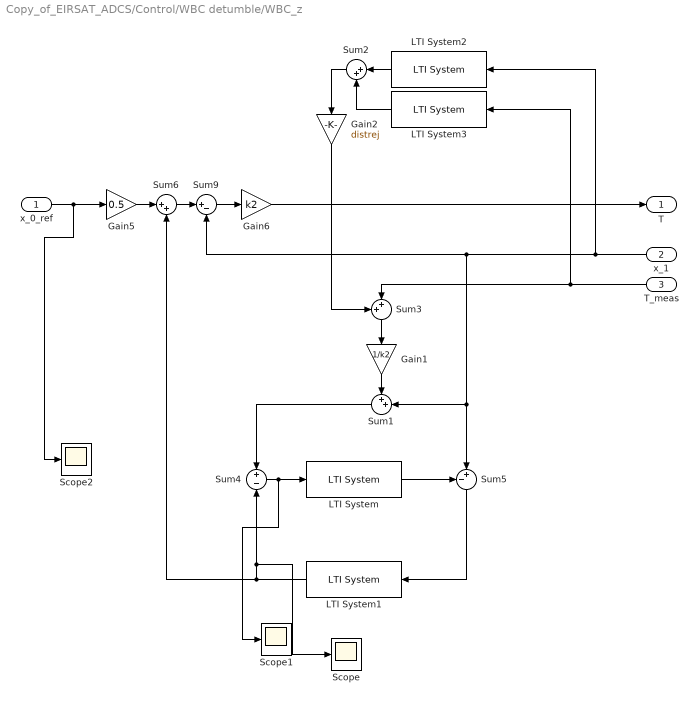
== system Copy_of_EIRSAT_ADCS/Control/WBC detumble/WBC_z ==
  x_0_ref : Inport
  x_1 : Inport  Port=2
  T_meas : Inport  Port=3
  Gain1 : Gain  Gain=1/k2
  Gain2 : Gain  Gain=distrej
  Gain5 : Gain  Gain=0.5
  Gain6 : Gain  Gain=k2
  LTI System : cstblocks/LTI System  sys=G2  IC=[]
  LTI System1 : cstblocks/LTI System  sys=G2  IC=[]
  LTI System2 : cstblocks/LTI System  sys=adr2(1)  IC=[]
  LTI System3 : cstblocks/LTI System  sys=adr2(2)  IC=[]
  Scope : Scope
  Scope1 : Scope
  Scope2 : Scope
  Sum1 : Sum  Inputs=++|
  Sum2 : Sum  Inputs=|++
  Sum3 : Sum  Inputs=++|
  Sum4 : Sum  Inputs=+|-
  Sum5 : Sum  Inputs=-+|
  Sum6 : Sum  Inputs=|++
  Sum9 : Sum  Inputs=|+-
  T : Outport
  wires:
  x_0_ref/1 -> Gain5/1, Scope2/1
  T_meas/1 -> LTI System3/1, Sum3/2
  Gain2/1 -> Sum3/1
  Sum3/1 -> Gain1/1
  Sum2/1 -> Gain2/1
  LTI System3/1 -> Sum2/2
  LTI System2/1 -> Sum2/1
  Sum6/1 -> Sum9/1
  Sum9/1 -> Gain6/1
  Gain6/1 -> T/1
  Gain5/1 -> Sum6/1
  LTI System1/1 -> Sum6/2, Sum4/2, Scope/1
  Sum4/1 -> LTI System/1, Scope1/1
  LTI System/1 -> Sum5/1
  Sum5/1 -> LTI System1/1
  x_1/1 -> LTI System2/1, Sum9/2, Sum5/2, Sum1/2
  Gain1/1 -> Sum1/1
  Sum1/1 -> Sum4/1

== system Copy_of_EIRSAT_ADCS/Control/no control/Bus ==
  In1 : Inport
  In2 : Inport  Port=2
  Bus Creator : BusCreator  Inputs=10
  Bus Selector1 : BusSelector  OutputSignals=omega_b_inert,qb_i,LongLatAlt,qb_o,qo_i,omega_orbit,T_ctrlr_meas,B_real,q_ref
  Out1 : Outport
  wires:
  In1/1 -> Bus Selector1/1
  Bus Creator/1 -> Out1/1
  Bus Selector1/1 -> Bus Creator/1  "<omega_b_inert>"
  Bus Selector1/2 -> Bus Creator/2  "<qb_i>"
  Bus Selector1/3 -> Bus Creator/3  "<LongLatAlt>"
  Bus Selector1/4 -> Bus Creator/4  "<qb_o>"
  Bus Selector1/5 -> Bus Creator/5  "<qo_i>"
  Bus Selector1/6 -> Bus Creator/6  "<omega_orbit>"
  Bus Selector1/7 -> Bus Creator/7  "<T_ctrlr_meas>"
  Bus Selector1/8 -> Bus Creator/8  "<B_real>"
  In2/1 -> Bus Creator/10  "T_ctrlr"
  Bus Selector1/9 -> Bus Creator/9  "<q_ref>"

== system Copy_of_EIRSAT_ADCS/Display/Change ref frame/q2RM1 ==
  In1 : Inport
  Add : Sum
  Constant : Constant  Value=eye(3)
  Fcn : Fcn  Commented=on  Expr=SkewSym([u(1),u(2),u(3)])
  Gain : Gain
  Interpreted MATLAB Function : MATLABFcn  MATLABFcn=SkewSym([u(1),u(2),u(3)],1)  OutputDimensions=9
  Math Function : Math  Operator=square  SaturateOnIntegerOverflow=on
  Product : Product
  Reshape : Reshape  OutputDimensionality=Customize  OutputDimensions=[3,3]
  Selector : Selector  InputPortWidth=4  Indices=[1]
  Selector1 : Selector  InputPortWidth=4  Indices=[2 3 4]
  Sum : Sum
  Out1 : Outport
  wires:
  In1/1 -> Selector/1, Selector1/1
  Reshape/1 -> Math Function/1, Product/2
  Selector/1 -> Product/1
  Selector1/1 -> Interpreted MATLAB Function/1
  Product/1 -> Sum/1
  Math Function/1 -> Sum/2
  Sum/1 -> Gain/1
  Gain/1 -> Add/2
  Constant/1 -> Add/1
  Add/1 -> Out1/1
  Interpreted MATLAB Function/1 -> Reshape/1

== system Copy_of_EIRSAT_ADCS/Display1/Change ref frame/q2RM1 ==
  In1 : Inport
  Add : Sum
  Constant : Constant  Value=eye(3)
  Gain : Gain
  Interpreted MATLAB Function : MATLABFcn  MATLABFcn=SkewSym([u(1),u(2),u(3)],1)  OutputDimensions=9
  Math Function : Math  Operator=square  SaturateOnIntegerOverflow=on
  Product : Product
  Reshape : Reshape  OutputDimensionality=Customize  OutputDimensions=[3,3]
  Selector : Selector  InputPortWidth=4  Indices=[1]
  Selector1 : Selector  InputPortWidth=4  Indices=[2 3 4]
  Sum : Sum
  Out1 : Outport
  wires:
  Interpreted MATLAB Function/1 -> Reshape/1
  Add/1 -> Out1/1
  Constant/1 -> Add/1
  Gain/1 -> Add/2
  Sum/1 -> Gain/1
  Math Function/1 -> Sum/2
  Product/1 -> Sum/1
  Selector1/1 -> Interpreted MATLAB Function/1
  Selector/1 -> Product/1
  Reshape/1 -> Product/2, Math Function/1
  In1/1 -> Selector1/1, Selector/1

== system Copy_of_EIRSAT_ADCS/Variant Subsystem/2 coil dipole/B vect from inert frm to body frm ==
  B_i : Inport
  q : Inport  Port=2
  Math Function2 : Math  Operator=transpose  SaturateOnIntegerOverflow=on
  Product : Product  Multiplication=Matrix(*)
  q2RM : Subsystem
  B_b : Outport
  wires:
  B_i/1 -> Product/2
  Product/1 -> B_b/1
  Math Function2/1 -> Product/1
  q/1 -> q2RM/1(In1)
  q2RM/1(Out1) -> Math Function2/1

== system Copy_of_EIRSAT_ADCS/Variant Subsystem/3 coil dipole/B vect from inert frm to body frm ==
  B_i : Inport
  q : Inport  Port=2
  Math Function2 : Math  Operator=transpose  SaturateOnIntegerOverflow=on
  Product : Product  Multiplication=Matrix(*)
  q2RM : Subsystem
  B_b : Outport
  wires:
  B_i/1 -> Product/2
  Product/1 -> B_b/1
  Math Function2/1 -> Product/1
  q/1 -> q2RM/1(In1)
  q2RM/1(Out1) -> Math Function2/1

== system Copy_of_EIRSAT_ADCS/Variant Subsystem/Three Axis MagTorq/B vect from inert frm to body frm ==
  q : Inport
  B_i : Inport  Port=2
  Math Function1 : Math  Operator=transpose  SaturateOnIntegerOverflow=on
  Product : Product  Multiplication=Matrix(*)
  q2RM2 : Subsystem
  B_b : Outport
  wires:
  q2RM2/1(Out1) -> Math Function1/1
  q/1 -> q2RM2/1(In1)
  Math Function1/1 -> Product/1
  Product/1 -> B_b/1
  B_i/1 -> Product/2

== system Copy_of_EIRSAT_ADCS/Variant Subsystem/Three Axis MagTorq/B vect from inert frm to body frm1 ==
  q : Inport
  B_i : Inport  Port=2
  Math Function1 : Math  Operator=transpose  SaturateOnIntegerOverflow=on
  Product1 : Product  Multiplication=Matrix(*)
  q2RM2 : Subsystem
  B_b : Outport
  wires:
  B_i/1 -> Product1/2
  Math Function1/1 -> Product1/1
  q/1 -> q2RM2/1(In1)
  q2RM2/1(Out1) -> Math Function1/1
  Product1/1 -> B_b/1

== system Copy_of_EIRSAT_ADCS/Control/PD Zenith/B vect from inert frm to body frm/q2RM2 ==
  In1 : Inport
  Add : Sum
  Constant : Constant  Value=eye(3)
  Fcn : Fcn  Commented=on  Expr=SkewSym([u(1),u(2),u(3)])
  Gain : Gain  Gain=2
  Interpreted MATLAB Function : MATLABFcn  MATLABFcn=SkewSym([u(1),u(2),u(3)],1)  OutputDimensions=9
  Math Function : Math  Operator=square  SaturateOnIntegerOverflow=on
  Product : Product
  Reshape : Reshape  OutputDimensionality=Customize  OutputDimensions=[3,3]
  Selector : Selector  InputPortWidth=4  Indices=[1]
  Selector1 : Selector  InputPortWidth=4  Indices=[2 3 4]
  Sum : Sum
  Out1 : Outport
  wires:
  Interpreted MATLAB Function/1 -> Reshape/1
  Add/1 -> Out1/1
  Constant/1 -> Add/1
  Gain/1 -> Add/2
  Sum/1 -> Gain/1
  Math Function/1 -> Sum/2
  Product/1 -> Sum/1
  Selector1/1 -> Interpreted MATLAB Function/1
  Selector/1 -> Product/1
  Reshape/1 -> Product/2, Math Function/1
  In1/1 -> Selector1/1, Selector/1
